simulink model "mconversion_nested_lib2"  (Simulink 6.1)
settings: Solver=FixedStepDiscrete  StartTime=0.0  StopTime=2  FixedStep=1  RelTol=1e-3
libraries: mconversion12aLib2 x1
settings Model: Creator=mshakeri  LastModifiedBy=mshakeri  ExtModeAutoUpdateStatusClock=off
settings DataIOCC: ExternalInput=utStr  SaveFormat=StructureWithTime  SaveState=on  SignalLoggingName=logsOut
settings OptimizationCC: InlineParams=on  InlineInvariantSignals=off  LifeSpan=1
settings DebuggingCC: CheckExecutionContextPreStartOutputMsg=on  CheckExecutionContextRuntimeOutputMsg=on
settings HardwareCC: TargetUnknown=on
settings RTWCC: SystemTargetFile=ert.tlc  TemplateMakefile=ert_default_tmf  RetainRTWFile=on  ProcessScript=ert_make_rtw_hook
settings ERTTargetCC: TargetFcnLib=ansi_tfl_tmw.mat  GenFloatMathFcnCalls=ANSI_C  GenerateSampleERTMain=on  SupportContinuousTime=on  SupportNonInlinedSFcns=on  ERTCustomFileTemplate=example_file_process.tlc  InitialValueSource=Model

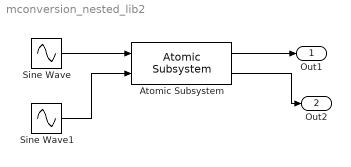
== system mconversion_nested_lib2 ==
  Atomic Subsystem : mconversion12aLib2/Atomic Subsystem
  Sine Wave : Sin  SampleTime=0
  Sine Wave1 : Sin  SampleTime=0
  Out1 : Outport
  Out2 : Outport  Port=2
  wires:
  Sine Wave/1 -> Atomic Subsystem/1
  Sine Wave1/1 -> Atomic Subsystem/2
  Atomic Subsystem/1 -> Out1/1
  Atomic Subsystem/2 -> Out2/1
